simulink model "VehRT_211219"  (R2019b)
settings: Solver=ode5  StartTime=0.0  StopTime=Inf  FixedStep=Ts  RelTol=1e-3  EnableMultiTasking=on
InitFcn:
  | VehRT_Init_211219;
  | Ts=0.0005;
values from neighbouring files (symbols this model uses):
  damping_p = 0.113    [VehRT_Init_211219.m]
  Ff_ab_p = 0.41    [VehRT_Init_211219.m]
  Ff_c_p = 0.4    [VehRT_Init_211219.m]
  friction_enable = 1    [VehRT_Init_211219.m]
  sigma0_p = 200    [VehRT_Init_211219.m]
  sigma1_p = (200)^0.5    (= 14.1421356237)    [VehRT_Init_211219.m]
  td = 0.01    [VehRT_Init_211219.m]
  theta_sb_p = 0.03    [VehRT_Init_211219.m]
undefined symbols (not defined in the file or in its folder): C, canChannel, D, DiscIntNeverNeededParam, g, IO306, Kf, Kr, Lf, Lr, M, magnitude, sigma, trajectory_x11_, trajectory_x12_, trajectory_x13_, trajectory_x14_, trajectory_x15_, trajectory_x16_, trajectory_x17_, trajectory_x21_, trajectory_x22_, trajectory_x23_, trajectory_x24_, trajectory_x25_, trajectory_x26_, trajectory_x27_, trajectory_y11_, trajectory_y12_, trajectory_y13_, trajectory_y14_, trajectory_y15_, trajectory_y16_, trajectory_y17_, trajectory_y21_, trajectory_y22_, trajectory_y23_, trajectory_y24_, trajectory_y25_, trajectory_y26_, trajectory_y27_, zeta
libraries: canmsglib x31, speedgoatlib_IO612 x20, slrtlib x15, simulink x5, speedgoatlib_IO133 x3, xpcutilitieslib x2, canlib x2, xpcrtudplib x2, speedgoatlib_fpga x1, speedgoatlib_fpga_dio x1, autolibshared x1, speedgoatlib_fpga_quadrature x1
(part 4 of 4)

== matlab function VehRT_211219/CEC Vehicle Dynamics 2021/CEC Vehicle Model 2021/Tires ==
  data: X input size=6; S input size=8; T_d input double size=4; I_drv input; T_b input; mu input double size=4; Fzs input; X_dot output double size=6; S_dot output double size=8; wg0 output; Ag0 output; uw input size=4; vw input size=4; Fwx output double size=4; Fwy output double size=4; delta input size=2; Mwz output double size=4; kw0 output; chamber input
% 轮胎模型（carsim_215_55_r17）
% V0.0.3 20211001 xiataokai 修改回正力跳变问题
% V0.0.4 20211008 xiataokai 加入更多状态维度

function [X_dot, S_dot, wg0, Ag0, Fwx, Fwy, Mwz ,kw0] = tir(X, S, T_d, I_drv, T_b, mu, Fzs, uw, vw, delta, chamber)
% delta的单位是rad
% Effective roling radius, m
Rw = 0.325; 
% Tire inertial, kg*m^2
Iw = 1.5; 
% Tire camber angle, deg
gamma0 = 0;
% Tire Rolling Resistance1, -
Rr_c = 0.0038; 
% Tire Rolling Resistance2, s/m
Rr_v = 0.000026/3.6; 
% Minimum tire logitudinal speed for slip calculation CTM(29), m/s 
Vmin = 0.5/3.6; 
% Relaxation length for lateral slip, m
Ly = 0.5; 
% Relaxation length for logitudinal slip, m
Lx = 0.5; 

% Differential shaft to left wheel intertial, kg-m2
Diff_IL = 0.009;
% Differential shaft to right wheel intertial, kg-m2
Diff_IR = 0.009;

% Slip rate and slip angle
k1 = Rw*X(1)/max(abs(uw(1)),Vmin)-1;
k2 = Rw*X(2)/max(abs(uw(2)),Vmin)-1;
k3 = Rw*X(3)/max(abs(uw(3)),Vmin)-1;
k4 = Rw*X(4)/max(abs(uw(4)),Vmin)-1;
a1 = -atan(vw(1)/max(abs(uw(1)),Vmin)) + delta(1);  % 20210809符号问题，这里的轮胎侧偏角取负才是对的  
a2 = -atan(vw(2)/max(abs(uw(2)),Vmin)) + delta(2);
a3 = -atan(vw(3)/max(abs(uw(3)),Vmin));
a4 = -atan(vw(4)/max(abs(uw(4)),Vmin));

kw0 = zeros(4,1); kw0(1) = k1; kw0(2) = k2; kw0(3)= k3; kw0(4) = k4;

% Lagged slip rate and slip angle (Tire transients)
S_dot = zeros(8,1);
S_dot(1) = max(abs(uw(1)),Vmin)/Lx*(k1-S(1)); % CTM(28)
S_dot(2) = max(abs(uw(2)),Vmin)/Lx*(k2-S(2));
S_dot(3) = max(abs(uw(3)),Vmin)/Lx*(k3-S(3));
S_dot(4) = max(abs(uw(4)),Vmin)/Lx*(k4-S(4));
S_dot(5) = max(abs(uw(1)),Vmin)/Ly*(tan(a1)-S(5)); % CTM(27)
S_dot(6) = max(abs(uw(2)),Vmin)/Ly*(tan(a2)-S(6));
S_dot(7) = max(abs(uw(3)),Vmin)/Ly*(tan(a3)-S(7));
S_dot(8) = max(abs(uw(4)),Vmin)/Ly*(tan(a4)-S(8));

% Lateral force, longitudinal force, aligning torque
Fwx = zeros(4,1); Fwy = zeros(4,1); Mwz = zeros(4,1); 
[Fwx(1), Fwy(1), Mwz(1)] = carsim_215_55_r17(Fzs(1), S(1), atan(S(5))/pi*180, mu(1), chamber(1)*180/pi + gamma0);
[Fwx(2), Fwy(2), Mwz(2)] = carsim_215_55_r17(Fzs(2), S(2), atan(S(6))/pi*180, mu(2), chamber(2)*180/pi - gamma0);
[Fwx(3), Fwy(3), Mwz(3)] = carsim_215_55_r17(Fzs(3), S(3), atan(S(7))/pi*180, mu(3), gamma0);
[Fwx(4), Fwy(4), Mwz(4)] = carsim_215_55_r17(Fzs(4), S(4), atan(S(8))/pi*180, mu(4), -gamma0);

% Tire dynamics
X_dot = zeros(6,1);
M_LF = (-T_b(1)-Rw*Fwx(1)-0*Fzs(1)*Rw*(Rr_c+Rr_v*uw(1)));
M_RF = (-T_b(2)-Rw*Fwx(2)-0*Fzs(2)*Rw*(Rr_c+Rr_v*uw(2)));
X_dot(1) = (T_d(1) + M_LF + I_drv*(M_LF-M_RF)/(Iw+Diff_IL))/(Iw+Diff_IL+I_drv*(1+(Iw+Diff_IL)/(Iw+Diff_IR)));
X_dot(2) = (T_d(2) + M_RF + I_drv*(M_RF-M_LF)/(Iw+Diff_IL))/(Iw+Diff_IR+I_drv*(1+(Iw+Diff_IR)/(Iw+Diff_IL)));
X_dot(3) = (T_d(3)-T_b(3)-Rw*Fwx(3)-0*Fzs(3)*Rw*(Rr_c+Rr_v*uw(3)))/Iw;
X_dot(4) = (T_d(4)-T_b(4)-Rw*Fwx(4)-0*Fzs(4)*Rw*(Rr_c+Rr_v*uw(4)))/Iw;
X_dot(5) = X(1);
X_dot(6) = X(2);

% Information
wg0 = 0.5*(X(1)+X(2));
Ag0 = 0.5*(X(5)+X(6));
1;
end

function [Fx, Fy, Mz] = carsim_215_55_r17(Fz, k, a, mu, gamma)
% Magical formular model of the tires，fitted from CarSim 215/55 R17
% Fz(N) vertical load 
% k(0~1) slip rate
% a(deg) slip angle
% mu(0~1) friction coeeficient
% gamma(deg) camber angle
mu0 = 1;
Fz0 = 4.7807e+03;
PFxB0 = 22.1951;
PFxC0 = 1.3997;
PFxD0 = 4.6565e+03;
PFxE0 = 0.5490;
PFyB0 = 0.1390;
PFyC0 = 2.2067;
PFyD0 = 4.6603e+03;
PFyE0 = 1.0047;
PMzB0 = 0.2665;
PMzC0 = 2.1415;
PMzD0 = 72.4154;
PMzE0 = -6.9391;
PCFkappa0 = 15.3932*6.6204*Fz0*sin(2*atan(Fz0/6.6204/Fz0));
PCFalpha0 = 0.1535*5.5010*Fz0*sin(2*atan(Fz0/5.5010/Fz0));
PCMalpha0 = (0.0290*(Fz0/Fz0).^0.0530).*PCFalpha0;
PCFkappa = 15.3932*6.6204*Fz0*sin(2*atan(Fz/6.6204/Fz0));
PCFalpha = 0.1535*5.5010*Fz0*sin(2*atan(Fz/5.5010/Fz0));
PCMalpha = (0.0290*(Fz/Fz0).^0.0530).*PCFalpha;
PCFgamma = 0.010*Fz;
PCMgamma = 0.10*(0.07)^2/0.3*PCFkappa;  % 系数取值具体多少有待商榷，书上Table4.1给的0.3，这里改成0.10
% 横纵向联合全滑移
astar = a+PCFgamma/PCFalpha*gamma; %4.29
sx = k/(1.0+k+1e-7);
systar = tan(astar/180*pi)/(1.0+k+1e-7);
sstar = sqrt(sx^2+systar^2)+1e-7;
sxeq = sstar*sign(sx);
syeq = sstar*sign(systar);   % 这个sign参考了CarSim Tire_Models.pdf P34**
keq = sxeq/(1-sxeq+1e-7)*(PCFkappa/PCFkappa0)*(mu0/mu)*(Fz0/Fz);  % 这个式子用4.30还是4.30a有待考虑，这是4.30
aeq = atan(syeq)/pi*180*(PCFalpha/PCFalpha0)*(mu0/mu)*(Fz0/Fz);
% 横向力、纵向力、回正力计算
Fx = abs(sx/sstar)*(mu/mu0)*(Fz/Fz0)...
    *PFxD0*sin(PFxC0*atan(PFxB0*keq-PFxE0*(PFxB0*keq-atan(PFxB0*keq))));
Fy = abs(systar/sstar)*(mu/mu0)*(Fz/Fz0)...  % 这个abs与**的sign配套，不然Fx,Fy计算的符号不对了
    *PFyD0*sin(PFyC0*atan(PFyB0*aeq-PFyE0*(PFyB0*aeq-atan(PFyB0*aeq))));
Mzr = (PCMgamma+PCFgamma*PCMalpha/PCFalpha)./(1+100*(syeq).^2)*gamma/180*pi;  % 系数取值具体多少有待商榷
Mzcouple = -0.3*0.08*Fx*Fy/Fz0 - 0*0.08*Fx - 4*0.07*Fx*gamma/180*pi;  % 系数取值具体多少有待商榷
Mz = -abs(systar/sstar)*(mu/mu0)*(Fz/Fz0)*(PCMalpha/PCMalpha0)*(PCFalpha0/PCFalpha)...
    *PMzD0*sin(PMzC0*atan(PMzB0*aeq-PMzE0*(PMzB0*aeq-atan(PMzB0*aeq))))...
    +Mzr+Mzcouple;
1;
end

== matlab function VehRT_211219/CEC Vehicle Dynamics 2021/CEC Vehicle Model 2021/Vehicle Body ==
  settings: updateMethod=DISCRETE
  data: X input; Fwx input; Fwy input; Mwz input; delta input; X_dot output; Fzs output; uw output; vw output; delta output; u output; v output; Vyaw output; Vroll output; PX output; PY output; Pyaw output; Proll output
% 车身模型（仅X、Y、侧倾，无俯仰，要求全平直路面）
% V0.0.2 20211008 xiataokai 垂向力计算

function [X_dot, Fzs, uw, vw, delta, u, v, Vyaw, Vroll, PX, PY, Pyaw, Proll] = veh(X, Fwx, Fwy, Mwz, delta)
% sta的单位是deg
% The sprung mass of the vehicle, kg
ms = 1110 + 100 ; 
% The total mass of the vehicle, kg
m = ms + 71.4 + 54.5; 
% Vehicle roll inertia, kg*m^2 
Ix = 440.6 +1850*0.48^2; %  
% Vehicle yaw inertia, kg*m^2
Iz = 1343.1; 
% The arm length of the rolling, m
h = 0.31; 
% The height of the CoG, m
h_cg = 0.54; 
% Front axle distance to CoG, m
La = 1.04; 
% Rear axle distance to CoG, m
Lb = 1.56; 
% Axle distance, m
L = La+Lb; 
% Front wheel base, m
Wf = 1.48; 
% Rear wheel base, m
Wr = 1.485; 
% Front roll stiffness Nm/rad
Kf = 44000; 
% Rear roll stiffness, Nm/rad
Kr = 44000; 
% Front roll damping, Nm/rad/s
Df = 5000; 
% Rear roll damping, Nm/rad/s
Dr = 5000; 
% The air density, kg/m^3
rou = 1.225; 
% Drag coeeficient, -
Cx = 0.28; 
% Down force coeeficient, -
Cz = 0.18; 
% Cross-section area, m^2
Ar = 2.80; 
% Aero balance distribution coefficient, -
epsilon = 0.5; 
% The gravitational constant, kg*m/s^2
g = 9.80; 

% Vertical load initialization
persistent Fz
if isempty(Fz)
    Fz = [Lb/L,Lb/L,La/L,La/L]*m*g/2;  
end

% Aero dynamics
Fair_x = 0.5*Cx*rou*Ar*X(3)^2;
Fair_z = 0.5*Cz*rou*Ar*X(3)^2;

% Steering dynamics
delta1 = delta(1); delta2 = delta(1);
kFx = 1; kFy = 1;
Fx1 = (cos(delta1)*Fwx(1)*kFx-sin(delta1)*Fwy(1)*kFy);
Fy1 = (sin(delta1)*Fwx(1)*kFx+cos(delta1)*Fwy(1)*kFy);
Fx2 = (cos(delta2)*Fwx(2)*kFx-sin(delta2)*Fwy(2)*kFy);
Fy2 = (sin(delta2)*Fwx(2)*kFx+cos(delta2)*Fwy(2)*kFy);
Fx3 = Fwx(3)*kFx; Fy3 = Fwy(3)*kFy; Fx4 = Fwx(4)*kFx; Fy4 = Fwy(4)*kFy;

% Suspension dynamics
Mpsi_f = -Df*X(6)-Kf*X(5);
Mpsi_r = -Dr*X(6)-Kr*X(5);
Mx = ms*g*h*X(5) + Mpsi_f + Mpsi_r;
Fx_sum = Fx1+Fx2+Fx3+Fx4;
Fy_sum = Fy1+Fy2+Fy3+Fy4;
Mz_sum = 0.5*Wf*(Fx2-Fx1)+0.5*Wr*(Fx4-Fx3)+La*(Fy1+Fy2)-Lb*(Fy3+Fy4) ;


% Non-linear state space function of the vehicle dynamic
X_dot = zeros(8,1);
X_dot(1) = X(2);
X_dot(2) = Mz_sum/Iz; 
X_dot(3) = (Fx_sum-Fair_x)/m + X(2)*X(4) + ms*h/m*X(2)*X(5); % 211209 +ms...
X_dot(4) = (Fy_sum*Ix-ms*h*Mx)/(m*Ix-ms^2*h^2) - X(2)*X(3); %211209 -ms*h...不一致
X_dot(5) = X(6);
X_dot(6) = (-Fy_sum*ms*h+m*Mx)/(m*Ix-ms^2*h^2); %211209 -Fy_sum 不一致
X_dot(7) = X(3)*cos(X(1))-X(4)*sin(X(1));
X_dot(8) = X(3)*sin(X(1))+X(4)*cos(X(1));

%outputs
Fzs = zeros(4,1); Fzs(1) = Fz(1); Fzs(2) = Fz(2); Fzs(3) = Fz(3); Fzs(4) = Fz(4);
u = X(3);
v = X(4);
PX = X(7);
PY = X(8);
Pyaw = X(1);
Vyaw = X(2);
Proll = X(5);
Vroll = X(6);
uw = zeros(4,1);
uw(1) = X(3)-0.5*Wf*X(2); uw(2) = X(3)+0.5*Wf*X(2); 
uw(3) = X(3)-0.5*Wr*X(2); uw(4) = X(3)+0.5*Wr*X(2);
vw = zeros(4,1);
vw(1) = X(4)+La*X(2); vw(2) = X(4)+La*X(2); 
vw(3) = X(4)-Lb*X(2); vw(4) = X(4)-Lb*X(2);
%   %211209添加
% uw(1) = cos(delta1)*uw(1) + sin(delta1)*vw(1);
% vw(1) = cos(delta1)*vw(1) - sin(delta1)*uw(1);
% uw(2) = cos(delta2)*uw(2) + sin(delta2)*vw(2);
% vw(2) = cos(delta2)*vw(2) - sin(delta2)*uw(2);
% delta = [delta1; delta2];


% Tire vertical loads
Finer_x = m*(X_dot(3)-X(2)*X(4)) - ms*h*X(2)*X(5); % 211209 -ms*
Finer_y = m*(X_dot(4)+X(2)*X(3)) + ms*h*X_dot(6); % 211209 +ms*
Fz(1) = m*g/2*Lb/L + epsilon/2*Fair_z - Finer_x*h_cg/2/L - Finer_y*Lb*h_cg/L/Wf + Mpsi_f/Wf;
Fz(2) = m*g/2*Lb/L + epsilon/2*Fair_z - Finer_x*h_cg/2/L + Finer_y*Lb*h_cg/L/Wf - Mpsi_f/Wf;
Fz(3) = m*g/2*La/L + (1-epsilon)/2*Fair_z + Finer_x*h_cg/2/L - Finer_y*La*h_cg/L/Wr + Mpsi_r/Wf;
Fz(4) = m*g/2*La/L + (1-epsilon)/2*Fair_z + Finer_x*h_cg/2/L + Finer_y*La*h_cg/L/Wr - Mpsi_r/Wf;
end

== matlab function VehRT_211219/CEC Vehicle Dynamics 2021/CEC Vehicle Model 2021/Vehicle_initializer/MATLAB Function ==
  data: V input; gearInit output; vehXInit output; pwrXInit output; tirXInit output
% 车辆状态初始化
% V0.0.3 20211219 xiataokai 修改发动机怠速初始化
function [gearInit, vehXInit, pwrXInit, tirXInit] = init(V)
% Transmission gear ratio, - (gear1 ~ gear6)
Trans1_N = [3.538, 2.060, 1.404, 1.000, 0.713, 0.582];
% Transmission inertia, kg-m2 (gear1 ~ gear6)
Trans1_I = [0.037, 0.034, 0.042, 0.040, 0.040, 0.040];
% Transmission efficiency when driving, - (gear1 ~ gear6)
Trans1_ed = [0.920, 0.920, 0.950, 0.950, 0.980, 0.990];
% Transmission efficiency when coasting, - (gear1 ~ gear6)
Trans1_ec = [0.920, 0.920, 0.950, 0.950, 0.980, 0.990];
% Transmission shift duration legacy, s
Trans1_legacy = 0.25;
% Transmission shift shedule 1-2 (- , rpm) (throttle , output speed in lower gear)
Trans1_u12 = [0, 874; 0.2, 874; 0.8, 1653; 1, 1653]; 
Trans1_d21 = [0. 699; 0.4, 699; 0.8, 1240; 1, 1240]; 
% Transmission shift shedule 2-3 (- , rpm) (throttle , output speed in lower gear)
Trans1_u23 = [0, 1282; 0.2, 1282; 0.8, 2840; 1, 2840];
Trans1_d32 = [0. 1026; 0.4, 1026; 0.8, 2130; 1, 2130];
% Transmission shift shedule 3-4 (- , rpm) (throttle , output speed in lower gear)
Trans1_u34 = [0, 1800; 0.2, 1800; 0.8, 4167; 1, 4167];
Trans1_d43 = [0. 1440; 0.4, 1440; 0.8, 3125; 1, 3125];
% Transmission shift shedule 4-5 (- , rpm) (throttle , output speed in lower gear)
Trans1_u45 = [0, 2525; 0.2, 2525; 0.8, 5850; 1, 5850];
Trans1_d54 = [0. 2020; 0.4, 2020; 0.8, 4388; 1, 4388];
% Transmission shift shedule 5-6 (- , rpm) (throttle , output speed in lower gear)
Trans1_u56 = [0, 3093; 0.2, 3093; 0.8, 8205; 1, 8205];
Trans1_d65 = [0. 2474; 0.4, 2474; 0.8, 6154; 1, 6154];
% Transmission shedule collection
Trans1_u = {Trans1_u12, Trans1_u23, Trans1_u34, Trans1_u45, Trans1_u56};
Trans1_d = {Trans1_d21, Trans1_d32, Trans1_d43, Trans1_d54, Trans1_d65};

% Effective roling radius, m
Rw = 0.325; 
% Differential gear ratio, -
Diff_N = 5.0; % 4.1

% Engine idle speed, rpm
Eng1_idel = 750; 

% Backward status estimation
% No-slip wheel speed
AgInit = 0;
wtInit = V/3.6/Rw;
wgInit = wtInit*Diff_N;
wgroutInit = wgInit;
for gearInit = 1:6
   if(gearInit < 6 && Trans1_u{gearInit}(1,2) >= wgroutInit/2/pi*60)
       break;
   end
end
NtransInit = Trans1_N(gearInit);
wtcoInit = wgroutInit*NtransInit;
weInit = max(wtcoInit, Eng1_idel/60*2*pi);

% Initial status output
vehXInit = [0; 0; V/3.6; 0; 0; 0; 0; 0];
pwrXInit = [weInit; AgInit; wgroutInit];
tirXInit = [wtInit; wtInit; wtInit; wtInit; 0; 0];
1;
end

== matlab function VehRT_211219/CEC Vehicle Dynamics 2021/CEC Vehicle Model 2021/awCal/atan_and_r2d ==
  data: u input; y output
function y = fcn(u)

y = atan(u)/pi*180;

== matlab function VehRT_211219/Hardware Interfaces/Shiftting Display/MATLAB Function ==
  data: gear input; out output
function out = dis(gear)
dis = [uint8(1),uint8(3),uint8(7),uint8(15),uint8(31),uint8(63),uint8(127),uint8(255)];
out = dis(min(max(gear,1),8));
end

== matlab function VehRT_211219/Hardware Interfaces/RPM Display/MATLAB Function ==
  data: rpm input; out output
function out = dis(rpm)
dis = [uint8(1),uint8(2),uint8(3),uint8(4),uint8(5),uint8(6),uint8(7),uint8(8)];
rpm_min = 0;
rpm_max = 6000;
rpm_round = ceil(min(max((rpm-rpm_min)/(rpm_max-rpm_min),0),1)*8);
out = dis(min(max(rpm_round,1),8));
end

== matlab function VehRT_211219/Lane Keeping Basic/Lane Keeping Assistance/signal processing/path_following ==
  settings: updateMethod=DISCRETE
  data: u input; Y output; w input; prex input; prey input; qulv output
function [Y, qulv] = fcn(u, w, prex, prey)
x_re = u(abs(u-prex)<20&abs(w-prey)<20);
y_re = w(abs(u-prex)<20&abs(w-prey)<20);
if max(x_re)-min(x_re) > max(y_re)-min(y_re)
    x0_ada = prex-5 : 0.01 : prex+5;
    y0_ada = interp1(x_re, y_re, x0_ada,'spline');
else
    y0_ada = prey+5 : -0.01 : prey-5;
    x0_ada = interp1(y_re, x_re, y0_ada,'spline');
end
[dis, num] = min((prex-x0_ada).^2 + (prey-y0_ada).^2);
vec_road = [x0_ada(num+1),y0_ada(num+1),0]-[x0_ada(num),y0_ada(num),0];
vec_driver = [prex,prey,0]-[x0_ada(num),y0_ada(num),0];
direction  = cross(vec_road,vec_driver);
Y=dis*sign(direction(3));
x1 = x0_ada(num-300);    x2 = x0_ada(num);    x3 = x0_ada(num+300);
y1 = y0_ada(num-300);    y2 = y0_ada(num);    y3 = y0_ada(num+300);
z1 = x2^2 + y2^2 - x1^2 - y1^2;
z2 = x3^2 + y3^2 - x1^2 - y1^2;
z3 = x3^2 + y3^2 - x2^2 - y2^2;
vec1 = [x2, y2, 0] - [x1, y1, 0];
vec2 = [x3, y3, 0] - [x2, y2, 0];
direction  = cross(vec1,vec2);
if direction(3) ~=0
A = [(x2-x1), (y2-y1); (x3-x1), (y3-y1); (x3-x2), (y3-y2)];
B = 0.5*[z1;  z2;  z3];
P0 = (A'*A)\A'*B;
R1 = sqrt( (P0(1) - x1)^2 + (P0(2) - y1)^2 );
R2 = sqrt( (P0(1) - x2)^2 + (P0(2) - y2)^2 );
R3 = sqrt( (P0(1) - x3)^2 + (P0(2) - y3)^2 );
R = (R1 + R2 + R3)/3;
qulv = 1/R*sign(direction(3));
else
    qulv = 0;
end
end
